simulink model "exp7"  (R2025b)
settings: Solver=VariableStepAuto  StartTime=0.0  StopTime=10.0  RelTol=1e-3
libraries: simulink_extras x1, simulink x1
settings Model: Creator=bharatsimhareddy  LastModifiedBy=SUBHASH

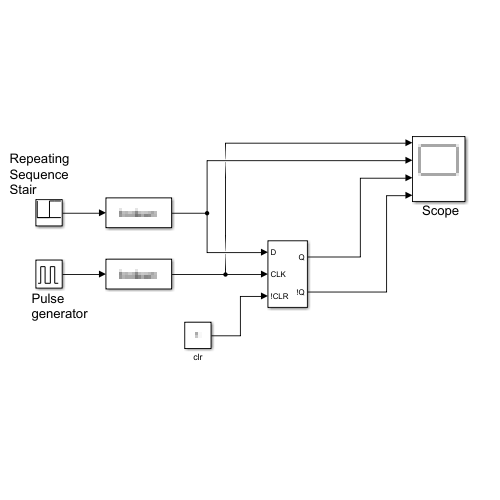
[thumbnail: Simulink's stored preview of the top-level diagram]
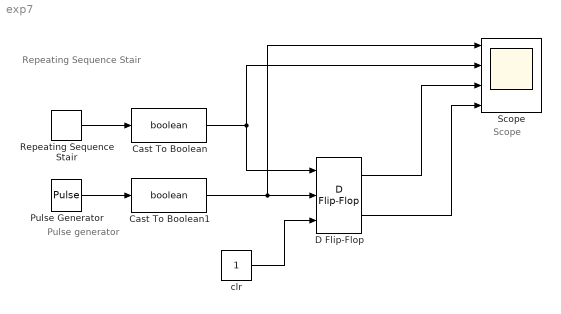
== system exp7 ==
  note: Repeating
      | Sequence
      | Stair
  note: Pulse generator
  note: Scope
  Cast To Boolean : DataTypeConversion  OutDataTypeStr=boolean  SaturateOnIntegerOverflow=off  RndMeth=Floor
  Cast To Boolean1 : DataTypeConversion  OutDataTypeStr=boolean  SaturateOnIntegerOverflow=off  RndMeth=Floor
  D Flip-Flop : simulink_extras/Flip Flops/D Flip-Flop
  Pulse Generator : DiscretePulseGenerator  PulseType=Time based  PulseWidth=50
  Repeating Sequence Stair : simulink/Sources/Repeating Sequence Stair  OutValues=[0 0 1 1].'  tsamp=1  OutMin=[]  OutMax=[]  OutDataTypeStr=double  OutputDataTypeScalingMode=double  OutDataType=fixdt(0,8)  ConRadixGroup=Best Precision: Vector-wise  OutScaling=2^-12
  Scope : Scope  NumInputPorts=4
      settings: ActiveDisplayYMinimum=-0.12499999999999997  ActiveDisplayYMaximum=1.125
  clr : Constant
  wires:
  clr/1 -> D Flip-Flop/3
  D Flip-Flop/1 -> Scope/3
  D Flip-Flop/2 -> Scope/4
  Repeating Sequence Stair/1 -> Cast To Boolean/1
  Cast To Boolean/1 -> D Flip-Flop/1, Scope/2
  Pulse Generator/1 -> Cast To Boolean1/1
  Cast To Boolean1/1 -> Scope/1, D Flip-Flop/2
